simulink model "bpsk_model"  (R2017b)
settings: Solver=VariableStepAuto  StartTime=0.0  StopTime=10000  RelTol=1e-3
libraries: commdigbbndpm3 x2, commsequence2 x2, commrflib2 x2, commsync2 x2, commfilt2 x2, commrfcorlib x1, commchan3 x1, commseqgen3 x1, commsink2 x1, commrandsrc3 x1
settings Model: Creator=croft  LastModifiedBy=croft

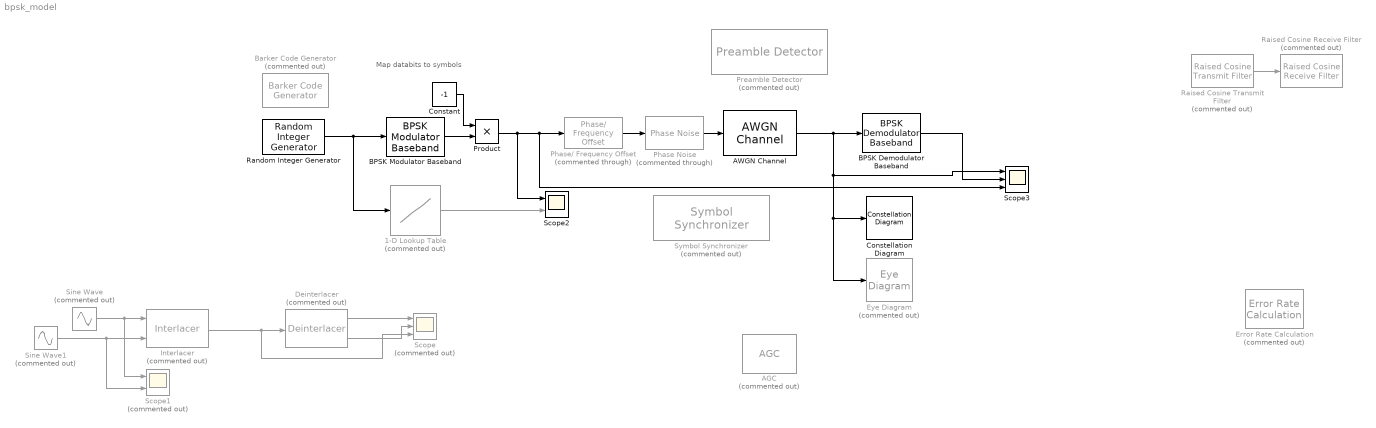
== system bpsk_model ==
  note: Map databits to symbols
  1-D Lookup Table : Lookup_n-D  Commented=on  NumberOfTableDimensions=1  BreakpointsForDimension1=[0 1]  Table=[-1 1]  InternalRulePriority=Speed  RndMeth=Simplest  InputSameDT=on
  AGC : commrfcorlib/AGC  Commented=on  LegacyMode=off  DetectorMethod=Rectifier  LoopMethod=Linear  UpdatePeriod=100  StepSize=0.1  AdaptationStepSize=0.01  DesiredOutputPower=1  AveragingLength=100  MaximumGain=30  MaxPowerGain=60  GainOutputPort=off  InputPowerOutputPort=off  SimulateUsing=Interpreted execution
      settings: SourceProductName=Communications System Toolbox
  AWGN Channel : commchan3/AWGN Channel  InputProcessing=Columns as channels (frame based)  seed=67  noiseMode="Signal to noise ratio  (SNR)"  EbNodB=10  EsNodB=10  SNRdB=10  bitsPerSym=1  Ps=1  Tsym=1  variance=1
  BPSK Demodulator Baseband : commdigbbndpm3/BPSK Demodulator Baseband  DecType=Hard decision  VarSource=Dialog  Variance=1  Ph=0  outDtype=Inherit via internal rule  derotateFactorWordLen=16  derotateFactorDataTypeStr=Inherit: Same word length as input  derotateFactorLastDataTypeStr=Inherit: Same word length as input
  BPSK Modulator Baseband : commdigbbndpm3/BPSK Modulator Baseband  Ph=0  outDtype=double  outWordLen=16  outUDDataType=sfix(16)  outFracLenMode=Best precision  outFracLen=15  outDataTypeStr=double  outLastDataTypeStr=double
  Barker Code Generator : commseqgen3/Barker Code Generator  Commented=on  Length=7  LengthSimulink=7  SampleTime=1  SamplesPerFrame=1  OutputDataType=double  SimulateUsing=Code generation
      settings: SourceProductName=Communications System Toolbox  SourceProductBaseCode=CM
  Constant : Constant  Value=-1
  Constellation Diagram : ConstellationDiagram
  Deinterlacer : commsequence2/Deinterlacer  Commented=on
      settings: SourceProductName=Communications System Toolbox  SourceProductBaseCode=CM
  Error Rate Calculation : commsink2/Error Rate Calculation  Commented=on  N=0  st_delay=0  cp_mode=Entire frame  subframe=[]  PMode=Workspace  WsName=ErrorVec  RsMode2=off  stop=off  numErr=100  maxBits=1e6
  Eye Diagram : EyeDiagram  Commented=on
  Interlacer : commsequence2/Interlacer  Commented=on
      settings: SourceProductName=Communications System Toolbox  SourceProductBaseCode=CM
  Phase Noise : commrflib2/Phase Noise  Commented=through  PhNs=[-60 -80]  Fo=[20 200]  Fs=1024  seed=2137
      settings: SourceProductName=Communications System Toolbox  SourceProductBaseCode=CM
  Phase/ Frequency Offset : commrflib2/Phase// Frequency Offset  Commented=through  phaseOffset=45  freqPort=off  freqOffset=1
      settings: SourceProductName=Communications System Toolbox
  Preamble Detector : commsync2/Preamble Detector  Commented=on  Input=Symbol  Preamble=[ 0;1;0;1]  Threshold=3  DetectionMetricOutput=off  Detections=All  SimulateUsing=Code generation
      settings: SourceProductName=Communications System Toolbox  SourceProductBaseCode=CM
  Product : Product
  Raised Cosine Receive Filter : commfilt2/Raised Cosine Receive Filter  Commented=on  filtType=Square root  R=0.2  filtSpan=10  N=8  downFactor=8  downOffset=0  filterGain=1  InputProcessing=Columns as channels (frame based)  RateOptions=Enforce single-rate processing  framing=Mute  checkCoeff=off  variableName=rcRxFilt  currentFiltSpan=10  D=5  inputOffset=0  sampMode=Mute  saveAsFlag=0  rateMode=Downsampling  checkGain=Normalized  launchFVT=on  roundingMode=Floor  overflowMode=off  coeffDataTypeStr=Inherit: Same word length as input  coeffMin=[]  coeffMax=[]  coeffLastDataTypeStr=Inherit: Same word length as input  accumDataTypeStr=Inherit: Same as product output  accumLastDataTypeStr=Inherit: Same as product output  outputDataTypeStr=Inherit: Same as accumulator  outputMin=[]  outputMax=[]  outputLastDataTypeStr=Inherit: Same as accumulator
  Raised Cosine Transmit Filter : commfilt2/Raised Cosine Transmit Filter  Commented=on  filtType=Square root  R=0.2  filtSpan=10  N=8  filterGain=1  InputProcessing=Columns as channels (frame based)  RateOptions=Enforce single-rate processing  framing=Mute  checkCoeff=off  variableName=rcTxFilt  checkGain=Normalized  sampMode=Mute  saveAsFlag=0  currentFiltSpan=10  D=(10)/2  launchFVT=on  roundingMode=Floor  overflowMode=off  coeffDataTypeStr=Inherit: Same word length as input  coeffMin=[]  coeffMax=[]  coeffLastDataTypeStr=Inherit: Same word length as input  outputDataTypeStr=Inherit: Same as accumulator  outputMin=[]  outputMax=[]  outputLastDataTypeStr=Inherit: Same as accumulator
  Random Integer Generator : commrandsrc3/Random Integer Generator  SetSize=2  SeedSource=Auto  Seed=0  SampleTime=1  SamplesPerFrame=1  OutputDataType=double  SimulateUsing=Code generation
  Scope : Scope  Commented=on  NumInputPorts=3
  Scope1 : Scope  Commented=on  NumInputPorts=2
  Scope2 : Scope  NumInputPorts=2
  Scope3 : Scope  NumInputPorts=3
  Sine Wave : Sin  Commented=on  SineType=Sample based  SampleTime=1/10
  Sine Wave1 : Sin  Commented=on  SineType=Sample based  SampleTime=1/10  Offset=2
  Symbol Synchronizer : commsync2/Symbol Synchronizer  Commented=on  Modulation=PAM/PSK/QAM  TimingErrorDetector=Zero-Crossing (decision-directed)  SamplesPerSymbol=2  DampingFactor=1  NormalizedLoopBandwidth=0.01  DetectorGain=2.7  TimingErrorOutputPort=on  SimulateUsing=Code generation
      settings: SourceProductName=Communications System Toolbox  SourceProductBaseCode=CM
  wires:
  Raised Cosine Transmit Filter/1 -> Raised Cosine Receive Filter/1
  Interlacer/1 -> Scope/3, Deinterlacer/1
  Deinterlacer/1 -> Scope/1
  Deinterlacer/2 -> Scope/2
  Sine Wave/1 -> Scope1/1, Interlacer/1
  Sine Wave1/1 -> Scope1/2, Interlacer/2
  Random Integer Generator/1 -> 1-D Lookup Table/1, BPSK Modulator Baseband/1
  BPSK Modulator Baseband/1 -> Product/2
  Constant/1 -> Product/1
  Product/1 -> Scope3/3, Phase/ Frequency Offset/1, Scope2/1
  AWGN Channel/1 -> BPSK Demodulator Baseband/1, Constellation Diagram/1, Eye Diagram/1, Scope3/1
  Phase Noise/1 -> AWGN Channel/1
  Phase/ Frequency Offset/1 -> Phase Noise/1
  1-D Lookup Table/1 -> Scope2/2
  BPSK Demodulator Baseband/1 -> Scope3/2
